simulink model "w1prob7"  (R2020a)
settings: Solver=VariableStepAuto  StartTime=0.0  StopTime=10.0  RelTol=1e-3
libraries: simulink x1
settings Model: Creator=Anjali123  LastModifiedBy=Anjali123

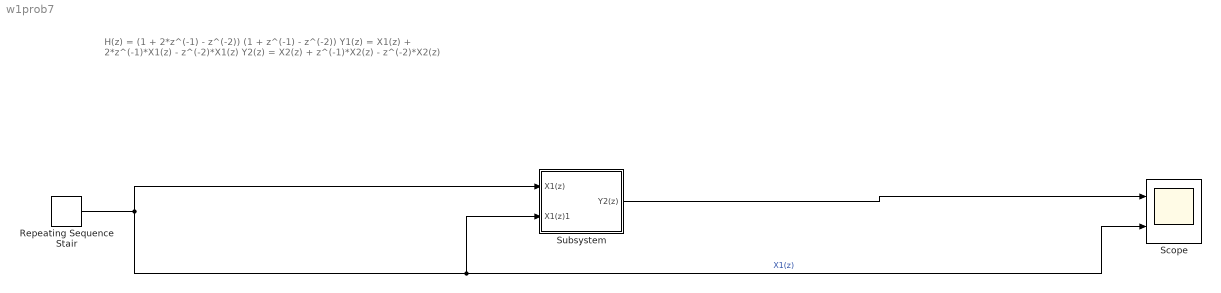
== system w1prob7 ==
  note: H(z) = (1 + 2*z^(-1) - z^(-2)) (1 + z^(-1) - z^(-2))
      | Y1(z) = X1(z) + 2*z^(-1)*X1(z) - z^(-2)*X1(z)
      | Y2(z) = X2(z) + z^(-1)*X2(z) - z^(-2)*X2(z)
  Repeating Sequence Stair : simulink/Sources/Repeating Sequence Stair  OutValues=[3 1 4 2 1].'  tsamp=0.1  OutMin=[]  OutMax=[]  OutDataTypeStr=double  OutputDataTypeScalingMode=double  OutDataType=fixdt(0,8)  ConRadixGroup=Best Precision: Vector-wise  OutScaling=2^-12
  Scope : Scope  NumInputPorts=2
  Subsystem : Subsystem
  wires:
  Repeating Sequence Stair/1 -> Subsystem/1(X1(z)), Subsystem/2(X1(z)1), Scope/2  "X1(z)"
  Subsystem/1(Y2(z)) -> Scope/1

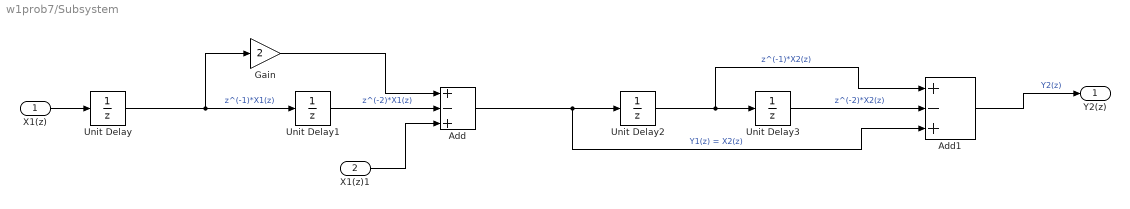
== system w1prob7/Subsystem ==
  X1(z) : Inport
  X1(z)1 : Inport  Port=2
  Add : Sum  Inputs=+-+
  Add1 : Sum  Inputs=+-+
  Gain : Gain  Gain=2
  Unit Delay{,1..3} (4 alike) : UnitDelay  SampleTime=-1  HasFrameUpgradeWarning=on
  Y2(z) : Outport
  wires:
  Add1/1 -> Y2(z)/1  "Y2(z)"
  Unit Delay2/1 -> Add1/1, Unit Delay3/1  "z^(-1)*X2(z)"
  Unit Delay1/1 -> Add/2  "z^(-2)*X1(z)"
  Add/1 -> Add1/3, Unit Delay2/1  "Y1(z) = X2(z)"
  Unit Delay/1 -> Gain/1, Unit Delay1/1  "z^(-1)*X1(z)"
  X1(z)1/1 -> Add/3
  Gain/1 -> Add/1
  X1(z)/1 -> Unit Delay/1
  Unit Delay3/1 -> Add1/2  "z^(-2)*X2(z)"
